simulink model "mainModelDOEJF"  (R2025a)
settings: Solver=VariableStepAuto  StartTime=0  StopTime=1000  RelTol=1e-3
undefined symbols (not defined in the file): advectiveCoefficientScale, AmbientTemperature, coolantTempSourceTemperatureScale, massCoolantScale, massModuleScale, scaledAdvectiveCoefficient, scaledCoolantTemp, scaledMassCoolant, scaledMassModule
libraries: fl_lib x265, nesl_utility x68, coolantFlow_lib x65, thermalCoupledCellResolution_lib x32, heatGenerationForCellResolvedModel x32, batt_lib x1, coolantFlowSwitch_lib x1
(part 1 of 4)
settings Model: Creator=jagmohanfanshal  LastModifiedBy=jagmohanfanshal
settings SimscapeCC: SimscapeLogType=all

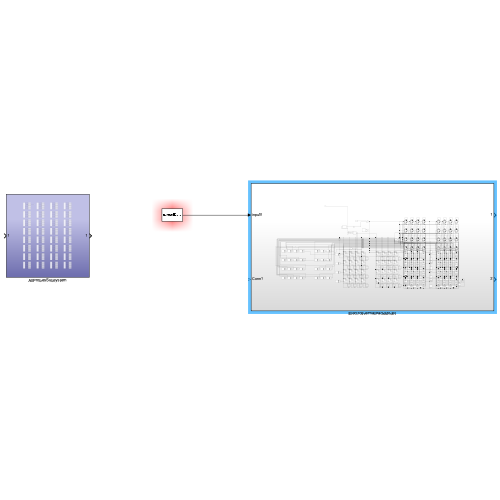
[thumbnail: Simulink's stored preview of the top-level diagram]
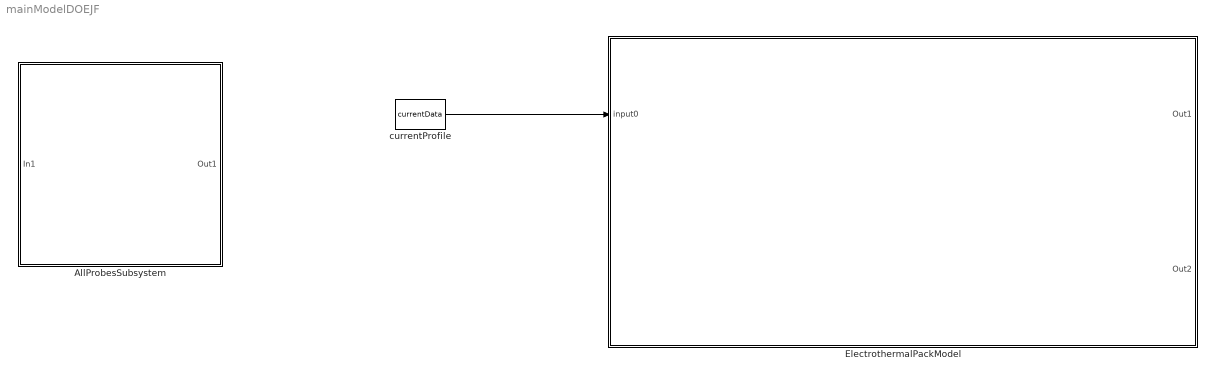
== system mainModelDOEJF ==
  AllProbesSubsystem : Subsystem
  ElectrothermalPackModel : Subsystem
  currentProfile : FromWorkspace  VariableName=currentData  SampleTime=10
  wires:
  currentProfile/1 -> ElectrothermalPackModel/1(input0)
